simulink model "vrbounce"  (R2019b)
settings: Solver=ode45  StartTime=0.0  StopTime=Inf  FixedStep=0.02  RelTol=1e-3
libraries: vrlib x2, instrumentlib x1
Description:
  | Bouncing Ball
  | 
  | The vrbounce example visualizes a ball bouncing from a floor. The ball deforms as it hits
  | the floor keeping the volume of the ball constant. The deformation is achieved by
  | modifying the scale field of the ball.
settings Model: EnablePacing=on  ExtModeTrigDuration=500  Creator=The MathWorks, Inc.  LastModifiedBy=onur
settings DataIOCC: SaveFormat=Array  SaveOutput=off  SaveTime=off  ReturnWorkspaceOutputs=off  SignalLoggingName=logsOut
settings OptimizationCC: BlockReduction=off  BooleanDataType=off  ExpressionDepthLimit=2147483647  InitFltsAndDblsToZero=on  LifeSpan=inf
settings DebuggingCC: UnderspecifiedInitializationDetection=Classic  MergeDetectMultiDrivingBlocksExec=none  CheckExecutionContextPreStartOutputMsg=on  CheckExecutionContextRuntimeOutputMsg=on  SignalResolutionControl=TryResolveAllWithWarning  MultiTaskDSMMsg=warning  MultiTaskCondExecSysMsg=none  FcnCallInpInsideContextMsg=warning  StateNameClashWarn=warning  SymbolicDimsDataTypeCodeGenerationDiagnostic=none  SFUnexpectedBacktrackingDiag=warning  SFNoUnconditionalDefaultTransitionDiag=warning  SFExecutionAtInitializationDiag=none  ArithmeticOperatorsInVariantConditions=warning
settings HardwareCC: ProdBitPerPointer=32  ProdBitPerSizeT=32  ProdBitPerPtrDiffT=32  ProdLargestAtomicFloat=None  ProdIntDivRoundTo=Undefined  ProdEndianess=Unspecified  ProdWordSize=32  ProdHWDeviceType=32-bit Generic  TargetUnknown=on
settings ModelReferenceCC: UpdateModelReferenceTargets=IfOutOfDate  PropagateSignalLabelsOutOfModel=off
settings SFSimCC: SimUseLocalCustomCode=off  CustomCodeUndefinedFunction=UseInterfaceOnly
settings RTWCC: RTWUseLocalCustomCode=off
settings CodeAppCC: StateflowObjectComments=on
settings GRTTargetCC: TargetFcnLib=ansi_tfl_tmw.mat  TargetLangStandard=C89/C90 (ANSI)  GeneratePreprocessorConditionals=Disable all  CombineOutputUpdateFcns=off  GRTInterface=on
settings ConfigComp: CovMetricSettings=d  CovHtmlReporting=on  CovSaveCumulativeToWorkspaceVar=on  CovSaveSingleToWorkspaceVar=on  CovExternalEMLEnable=off  CovSFcnEnable=off

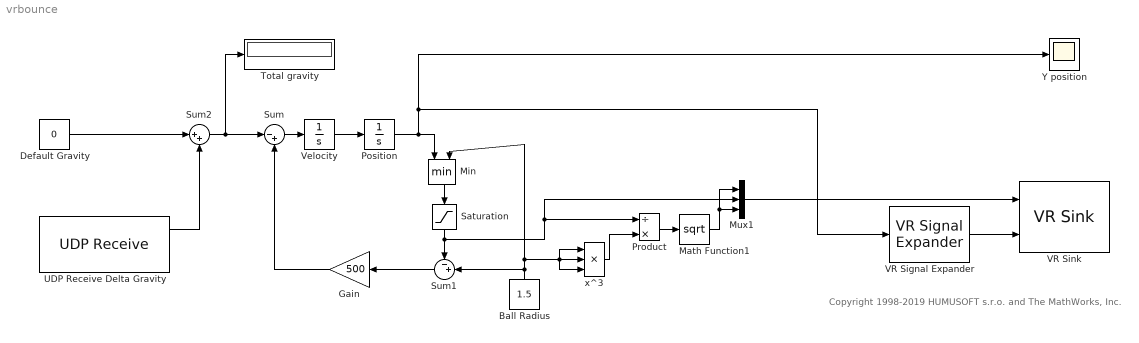
== system vrbounce ==
  note: Copyright 1998-2019 HUMUSOFT s.r.o. and The MathWorks, Inc.
  Ball Radius : Constant  Value=1.5
  Default Gravity : Constant  Value=0
  Gain : Gain  Gain=500  SaturateOnIntegerOverflow=on  OutDataTypeStr=Inherit: Same as input  ParamDataTypeStr=Inherit: Same as input
  Math Function1 : Math  Operator=sqrt  SaturateOnIntegerOverflow=on
  Min : MinMax  Inputs=2  ZeroCross=off  SaturateOnIntegerOverflow=on  InputSameDT=on
  Mux1 : Mux  Inputs=3
  Position : Integrator  InitialCondition=20  UpperSaturationLimit=Inf  LowerSaturationLimit=-Inf  ZeroCross=off
  Product : Product  Inputs=/*  SaturateOnIntegerOverflow=on  InputSameDT=on  OutDataTypeStr=Inherit: Same as first input
  Saturation : Saturate  UpperLimit=Inf  LowerLimit=1e-4  ZeroCross=off
  Sum : Sum  Inputs=|-+  SaturateOnIntegerOverflow=on  InputSameDT=on  OutDataTypeStr=Inherit: Same as first input
  Sum1 : Sum  Inputs=-+|  SaturateOnIntegerOverflow=on  InputSameDT=on  OutDataTypeStr=Inherit: Same as first input
  Sum2 : Sum  Inputs=|++  SaturateOnIntegerOverflow=on  InputSameDT=on  OutDataTypeStr=Inherit: Same as first input
  Total gravity : Display
  UDP Receive Delta Gravity : instrumentlib/UDP Receive  Host=localhost  Port=9090  LocalPort=8888  EnablePortSharing=off  GetLatestData=on  DataSize="[1  1]"  DataType=ASCII  ASCIIFormatting=%f  Terminator=LF  ByteOrder=LittleEndian  EnableBlockingMode=off  Timeout=10  SampleTime=0.01  LocalAddress=127.0.0.1
      settings: SourceProductName=Instrument Control Toolbox
  VR Signal Expander : vrlib/VR Signal Expander  outwidth=3  outidx=2
      settings: SourceProductName=Simulink
  VR Sink : vrlib/VR Sink  InstantiateOnLoad=on  SampleTime=0.02  ViewEnable=on  RemoteChange=off  RemoteView=off  FieldsWritten=Ball.scale.3.1.double#Ball.translation.3.1.double  WorldFileName=vrbounce.wrl  AutoView=on  VideoDimensions=[]  AllowVariableSize=off  FigureProperties="{'Position', 'Name', 'Viewpoint', 'CameraBound', 'CameraDirection', 'CameraPosition', 'CameraUpVector', 'ZoomFactor', 'Antialiasing', 'Headlight', 'Lighting', 'NavPanel', 'Sound', 'StatusBar', 'Stereo3D', 'Stereo3DCameraOffset', 'Stereo3DHIT', 'ToolBar', 'Textures', 'Transparency', 'Triad', 'Wireframe', 'NavZones', 'NavMode', 'NavSpeed', 'CaptureFileFormat', 'CaptureFileName', 'Record2DCompressMethod', 'Record2DCompressQuality', 'Record2D', 'Record2DFileName', 'Record2DFPS'; [5.0000000000000000e+00   9.2000000000000227e+01   4.2800000000000000e+02   2.7233333333333326e+02], 'VR Bouncing Ball', 'Ball', 'on', [0.0000000000000000e+00   0.0000000000000000e+00  -1.0000000000000000e+00], [0.0000000000000000e+00   0.0000000000000000e+00   0.0000000000000000e+00], [0.0000000000000000e+00   1.0000000000000000e+00   0.0000000000000000e+00], [1.0000000000000000e+00], 'on', 'on', 'on', 'halfbar', 'on', 'on', 'off', [1.0000000149011612e-01], [0.0000000000000000e+00], 'on', 'on', 'on', 'none', 'off', 'off', 'examine', 'normal', 'tif', '%f_anim_%n.tif', 'auto', [7.5000000000000000e+01], 'off', '%f_anim_%n.avi', 'auto'}"
      settings: SourceProductName=Simulink
  Velocity : Integrator  UpperSaturationLimit=Inf  LowerSaturationLimit=-Inf  ZeroCross=off
  Y position : Scope
  x^3 : Product  Inputs=3  SaturateOnIntegerOverflow=on  InputSameDT=on  OutDataTypeStr=Inherit: Same as first input
  wires:
  Velocity/1 -> Position/1
  Mux1/1 -> VR Sink/1
  VR Signal Expander/1 -> VR Sink/2
  Sum/1 -> Velocity/1
  Position/1 -> Min/1, Y position/1, VR Signal Expander/1
  Gain/1 -> Sum/2
  Min/1 -> Saturation/1
  Sum1/1 -> Gain/1
  Saturation/1 -> Sum1/1, Mux1/2, Product/1
  Product/1 -> Math Function1/1
  x^3/1 -> Product/2
  Math Function1/1 -> Mux1/1, Mux1/3
  Ball Radius/1 -> Sum1/2, Min/2, x^3/2, x^3/1, x^3/3
  Default Gravity/1 -> Sum2/1
  Sum2/1 -> Total gravity/1, Sum/1
  UDP Receive Delta Gravity/1 -> Sum2/2
